simulink model "Final_SAE_Without_PID"  (R2021a)
settings: Solver=VariableStepAuto  StartTime=0.0  StopTime=35  RelTol=1e-3
values from neighbouring files (symbols this model uses):
  B = 0.015    [Project_reading_1.m]
  C = 0.8    [Project_reading_1.m]
  g = 5    [Project_reading_1.m]
  J = 0.0236    [Project_reading_1.m]
  k = 3    [Project_reading_1.m]
  Ks = 18000    [Project_reading_1.m]
  Kt = 1.78    [Project_reading_1.m]
  L = 0.0063    [Project_reading_1.m]
  m = 8    [Project_reading_1.m]
  P = 1    [Project_reading_1.m]
  R = 2.1975    [Project_reading_1.m]
libraries: simulink_extras x2
settings Model: Creator=Panda  LastModifiedBy=Panda

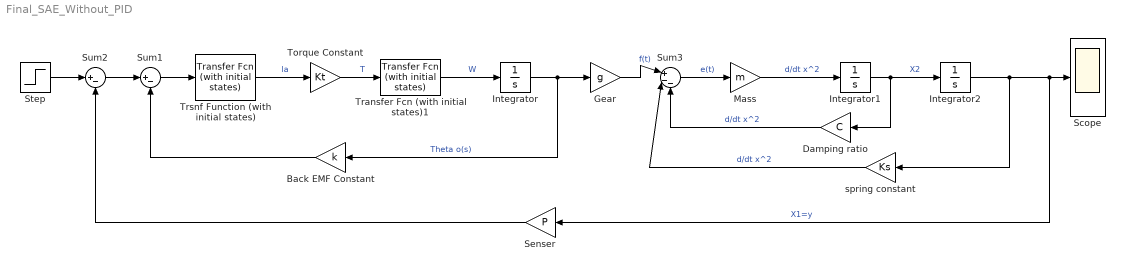
== system Final_SAE_Without_PID ==
  Back EMF Constant : Gain  Gain=k
  Damping ratio : Gain  Gain=C
  Gear : Gain  Gain=g
  Integrator : Integrator
  Integrator1 : Integrator
  Integrator2 : Integrator
  Mass : Gain  Gain=m
  Scope : Scope
  Senser : Gain  Gain=P
  Step : Step  SampleTime=0
  Sum1 : Sum  Inputs=|+-
  Sum2 : Sum  Inputs=|+-
  Sum3 : Sum  Inputs=|+--
  Torque Constant : Gain  Gain=Kt
  Transfer Fcn (with initial states)1 : simulink_extras/Additional Linear/Transfer Fcn (with initial states)  N=[1]  D="[J  B]"  X0=.5
  Trsnf Function (with initial states) : simulink_extras/Additional Linear/Transfer Fcn (with initial states)  N=[1]  D="[L  R]"  X0=.5
  spring constant : Gain  Gain=Ks
  wires:
  Back EMF Constant/1 -> Sum1/2
  Sum1/1 -> Trsnf Function (with initial states)/1
  Mass/1 -> Integrator1/1  "d/dt x^2"
  Torque Constant/1 -> Transfer Fcn (with initial states)1/1  "T"
  Trsnf Function (with initial states)/1 -> Torque Constant/1  "la"
  Sum3/1 -> Mass/1  "e(t)"
  Integrator/1 -> Back EMF Constant/1, Gear/1  "Theta o(s)"
  spring constant/1 -> Sum3/2  "d/dt x^2"
  Transfer Fcn (with initial states)1/1 -> Integrator/1  "W"
  Integrator2/1 -> Scope/1, Senser/1, spring constant/1  "X1=y"
  Integrator1/1 -> Integrator2/1, Damping ratio/1  "X2"
  Damping ratio/1 -> Sum3/3  "d/dt x^2"
  Gear/1 -> Sum3/1  "f(t)"
  Sum2/1 -> Sum1/1
  Step/1 -> Sum2/1
  Senser/1 -> Sum2/2
